simulink subsystem "Monitor"  (R2021b)
settings: Solver=VariableStepAuto  StartTime=0.0  StopTime=10.0  RelTol=1e-3
settings Model: Creator=DELL  LastModifiedBy=DELL

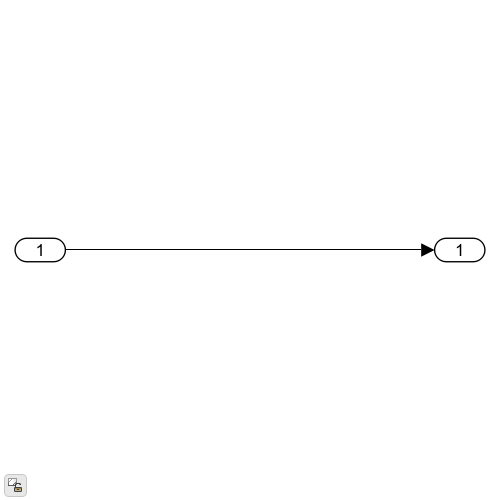
[thumbnail: Simulink's stored preview of the top-level diagram]
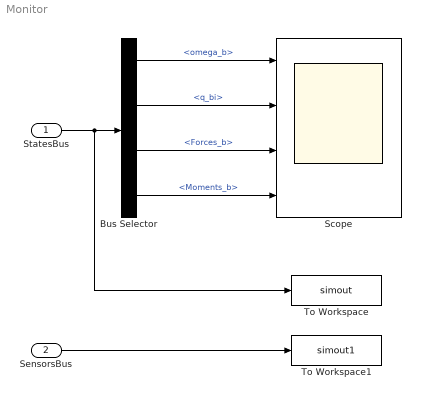
== system Monitor ==
  StatesBus : Inport
  SensorsBus : Inport  Port=2
  Bus Selector : BusSelector  OutputSignals=omega_b,q_bi,Forces_b,Moments_b
  Scope : Scope  NumInputPorts=4
  To Workspace : ToWorkspace  VariableName=simout  SaveFormat=Timeseries  SampleTime=-1
  To Workspace1 : ToWorkspace  VariableName=simout1  SaveFormat=Timeseries  SampleTime=-1
  wires:
  StatesBus/1 -> Bus Selector/1, To Workspace/1
  SensorsBus/1 -> To Workspace1/1
  Bus Selector/1 -> Scope/1  "<omega_b>"
  Bus Selector/2 -> Scope/2  "<q_bi>"
  Bus Selector/3 -> Scope/3  "<Forces_b>"
  Bus Selector/4 -> Scope/4  "<Moments_b>"
